simulink model "Pendulo2GDL"  (R2019b)
settings: Solver=VariableStepAuto  StartTime=0.0  StopTime=10.0  RelTol=1e-3
values from neighbouring files (symbols this model uses):
  b1 = c8    (= 0.01)    [PenduloDatos.m]
  b2 = c8    (= 0.01)    [PenduloDatos.m]
  g = 9.78    [PenduloDatos.m]
  I1 = 1/12*m1*(a1^2+d1^2)    (= 3.14166666667e-05)    [PenduloDatos.m]
  I2 = 1/12*m2*(a2^2+d2^2)    (= 1.20833333333e-05)    [PenduloDatos.m]
  l1 = c1    (= 0.3)    [PenduloDatos.m]
  lc1 = 0.25    [PenduloDatos.m]
  lc2 = 0.11    [PenduloDatos.m]
  m1 = c3    (= 0.065)    [PenduloDatos.m]
  m2 = c4    (= 0.025)    [PenduloDatos.m]
  XI = [0;0;0;0]    [PenduloDatos.m]
settings Model: Creator=javier  LastModifiedBy=ARQ SEVILLA R
settings DataIOCC: ReturnWorkspaceOutputs=off
settings DebuggingCC: ArithmeticOperatorsInVariantConditions=warning
settings SFSimCC: SimUseLocalCustomCode=off  CustomCodeUndefinedFunction=UseInterfaceOnly
settings RTWCC: RTWUseLocalCustomCode=off

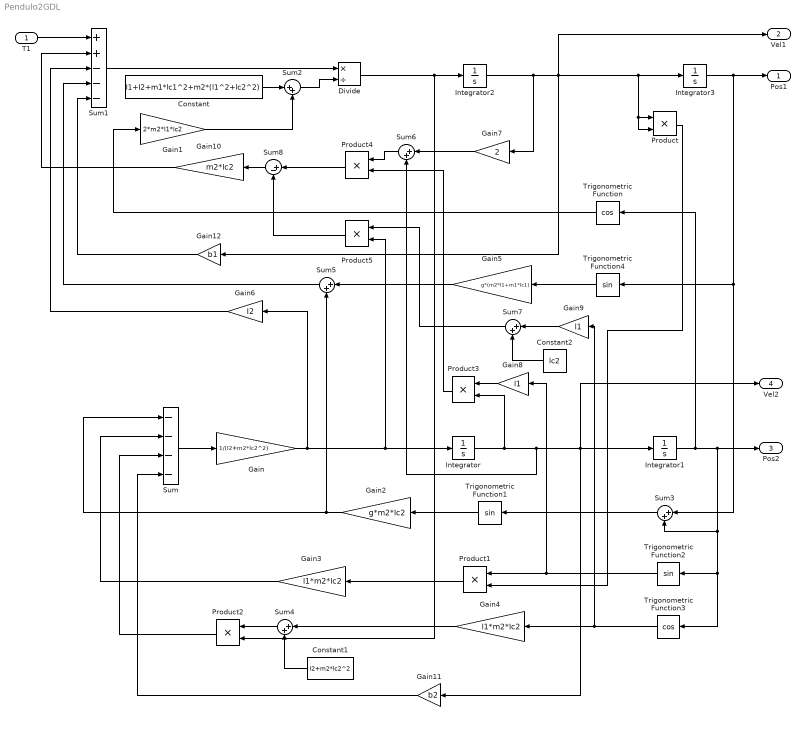
== system Pendulo2GDL ==
  T1 : Inport
  Constant : Constant  Value=I1+I2+m1*lc1^2+m2*(l1^2+lc2^2)
  Constant1 : Constant  Value=I2+m2*lc2^2
  Constant2 : Constant  Value=lc2
  Divide : Product  Inputs=*/
  Gain : Gain  Gain=1/(I2+m2*lc2^2)
  Gain1 : Gain  Gain=2*m2*l1*lc2
  Gain10 : Gain  Gain=m2*lc2
  Gain11 : Gain  Gain=b2
  Gain12 : Gain  Gain=b1
  Gain2 : Gain  Gain=g*m2*lc2
  Gain3 : Gain  Gain=l1*m2*lc2
  Gain4 : Gain  Gain=l1*m2*lc2
  Gain5 : Gain  Gain=g*(m2*l1+m1*lc1)
  Gain6 : Gain  Gain=I2
  Gain7 : Gain  Gain=2
  Gain8 : Gain  Gain=l1
  Gain9 : Gain  Gain=l1
  Integrator : Integrator  InitialCondition=XI(4)
  Integrator1 : Integrator  InitialCondition=XI(3)
  Integrator2 : Integrator  InitialCondition=XI(2)
  Integrator3 : Integrator  InitialCondition=XI(1)
  Product{,1..5} (6 alike) : Product
  Sum : Sum  Inputs=----
  Sum1 : Sum  Inputs=++---
  Sum{2..7} (6 alike) : Sum  Inputs=|++
  Sum8 : Sum  Inputs=|+-
  Trigonometric Function : Trigonometry  Operator=cos
  Trigonometric Function1 : Trigonometry
  Trigonometric Function2 : Trigonometry
  Trigonometric Function3 : Trigonometry  Operator=cos
  Trigonometric Function4 : Trigonometry
  Pos1 : Outport  VectorParamsAs1DForOutWhenUnconnected=off
  Vel1 : Outport  Port=2  VectorParamsAs1DForOutWhenUnconnected=off
  Pos2 : Outport  Port=3  VectorParamsAs1DForOutWhenUnconnected=off
  Vel2 : Outport  Port=4  VectorParamsAs1DForOutWhenUnconnected=off
  wires:
  Integrator1/1 -> Trigonometric Function/1, Trigonometric Function3/1, Trigonometric Function2/1, Sum3/2, Pos2/1
  Product4/1 -> Sum8/1
  Gain8/1 -> Product3/1
  Gain6/1 -> Sum1/3
  Sum7/1 -> Product5/1
  Sum1/1 -> Divide/1
  Gain10/1 -> Sum1/2
  Gain7/1 -> Sum6/1
  Trigonometric Function4/1 -> Gain5/1
  Sum5/1 -> Sum1/4
  Product2/1 -> Sum/3
  Sum8/1 -> Gain10/1
  Integrator3/1 -> Pos1/1, Sum3/1, Trigonometric Function4/1
  Gain1/1 -> Sum2/2
  Trigonometric Function3/1 -> Gain9/1, Gain4/1
  Integrator/1 -> Product3/2, Vel2/1, Integrator1/1, Gain11/1, Sum6/2
  Gain4/1 -> Sum4/1
  Sum4/1 -> Product2/1
  Gain2/1 -> Sum5/2, Sum/1
  Divide/1 -> Product2/2, Integrator2/1
  Constant/1 -> Sum2/1
  Sum/1 -> Gain/1
  Product/1 -> Product1/2
  Gain3/1 -> Sum/2
  Product1/1 -> Gain3/1
  Constant2/1 -> Sum7/2
  Constant1/1 -> Sum4/2
  Sum6/1 -> Product4/1
  Product5/1 -> Sum8/2
  Integrator2/1 -> Gain7/1, Vel1/1, Gain12/1, Product/2, Product/1, Integrator3/1
  Gain5/1 -> Sum5/1
  Trigonometric Function1/1 -> Gain2/1
  Trigonometric Function2/1 -> Gain8/1, Product1/1
  Trigonometric Function/1 -> Gain1/1
  T1/1 -> Sum1/1
  Sum3/1 -> Trigonometric Function1/1
  Sum2/1 -> Divide/2
  Gain/1 -> Product5/2, Integrator/1, Gain6/1
  Product3/1 -> Product4/2
  Gain9/1 -> Sum7/1
  Gain11/1 -> Sum/4
  Gain12/1 -> Sum1/5
